simulink model "Control_Law_1e"  (R2020b)
settings: Solver=FixedStepDiscrete  StartTime=0.0  StopTime=60  FixedStep=dt  RelTol=1e-3
InitFcn:
  | clear
  | clc
  | 
  | dtsim = 0.1;
  | dt =0.005;
  | dtdata = 0.01;
  | dtcontrol = 0.01;
  | 
  | I = [1.01560749 0.00028915 0.00002257; 0.00028915 0.17343628 0.00936307; 0.00002257 0.00936307 1.01561864];
  | 
  | Iinv = I^-1;
  | 
  | % Reaction Wheels
  | 
  | x = cosd(70);
  | y = sqrt(0.5*(1^2-x^2));
  | e1 = [x;y;y];
  | e2 = [x;-y;y];
  | e3 = [x;-y;-y];
  | e4 = [x;y;-y];
  | %e1 = [y;x;y];
  | %e2 = [-y;x;y];
  | %e3 = [-y;-x;y];
  | %e4 = [y;-x;y];
  | e = [e1 e2 e3 e4];
  | 
  | %Reaction Wheels MOI and Ang Vel
  | 
  | Irw = 0.000453158;
  | 
  | w1 =1500*2*pi/60;
  | w2 = 1500*2*pi/60;
  | w3 = -1500*2*pi/60;
  | w4 = -1500*2*pi/60;
  | 
  | alpha_max = 1537.9; %rad/sec^2
  | 
  | Tmax = Irw*alpha_max; % Irw*alpha_max;
  | 
  | %User Input Check
  | 
  | Rt = 170*pi/180;
  | Pt = 10*pi/180;
  | Yt = 170*pi/180;
  | 
  | if Pt > 20*pi/180
  | 
  | error('Input a pitch angle lower that 20 degrees')
  | 
  | end
  | 
  | RPYtarget = [Rt;Pt;Yt];
  | 
  | q_target = [cos(Rt/2)*cos(Pt/2)*cos(Yt/2) -  sin(Rt/2)*sin(Pt/2)*sin(Yt/2);
  |                   sin(Rt/2)*cos(Pt/2)*cos(Yt/2) + cos(Rt/2)*sin(Pt/2)*sin(Yt/2);
  |                  cos(Rt/2)*sin(Pt/2)*cos(Yt/2) -   sin(Rt/2)*cos(Pt/2)*sin(Yt/2);
  |                  cos(Rt/2)*cos(Pt/2)*sin(Yt/2) +  sin(Rt/2)*sin(Pt/2)*cos(Yt/2)];
  | 
  | % Inital Conditions
  | 
  | wo = [0;0;0];
  | ro = [6378;0;0];
  | romag = 6378;
  | mu = 398600;
  | vo = sqrt(mu/romag)*[0;1;0];
  | ho = [0;0;0];
  | 
  | a = 6378;
  | n = sqrt(mu/a^3);
  | 
  | %k1 = (4-2)/3;
  | %k2 = (I(3,3) - I(1,1))/I(2,2);
  | %k3  = (I(2,2) - I(1,1))/I(3,3);
  | 
  | k1 = (I(2,2) - I(3,3))/I(1,1);
  | k2 = (I(2,2) - I(3,3))/I(2,2);
  | k3 = (I(2,2) - I(1,1))/I(3,3);
  | 
  | F = -2*n^2*[4*k1, 0, 0;0, 3*k2, 0; 0, 0, k3];
  | G = n*[0 0 (1-k1);0 0 0;(k3-1) 0 0 ];
  | 
  | Iinv =[1/I(1,1) 0 0; 0 1/I(2,2) 0; 0 0 1/I(3,3)];
  | 
  | A = [zeros(3,3) 0.5*eye(3);F G];
  | B = [zeros(3,3); Iinv];
  | R = eye(3);
  | Rinv = R^-1;
  | 
  | Q_nominal= diag([1,1,1,10,10,10]);
  | S_nominal = icare(A,B,Q_nominal,R);
  | K_nominal = -Rinv*B'*S_nominal;
  | 
  | Q_corrective= diag([1,1,1,10,10,10]);
  | S_corrective = icare(A,B,Q_corrective,R);
  | K_corrective = -Rinv*B'*S_corrective;
  | 
  | Q_yawsweep= diag([1,1,1,10,15,10]);
  | S_yawsweep = icare(A,B,Q_yawsweep,R);
  | K_yawsweep = -Rinv*B'*S_yawsweep;
  | 
  | %Initial Attitude
  | 
  | R = 0*pi/180;
  | P = 0*pi/180;
  | Y =0*pi/180;
  | 
  | RPY = [R; P; Y];
  | 
  | qo = [cos(R/2)*cos(P/2)*cos(Y/2) - sin(R/2)*sin(P/2)*sin(Y/2);
  |          sin(R/2)*cos(P/2)*cos(Y/2) + cos(R/2)*sin(P/2)*sin(Y/2);
  |          cos(R/2)*sin(P/2)*cos(Y/2) - sin(R/2)*cos(P/2)*sin(Y/2);
  |          cos(R/2)*cos(P/2)*sin(Y/2) + sin(R/2)*sin(P/2)*cos(Y/2)];
  | 
  | %Visual Int
  | 
  | myworld = vrworld('SimulinkTest.wrl');
  | open(myworld);
  | 
  | set(0,'Units','pixels');
  | scnsize = get(0,'ScreenSize');
  | 
  | f1 = vrfigure(myworld,scnsize);
StopFcn:
  | close all
  | 
  | %Set default grid axes to be on
  | set(groot,'defaultAxesXGrid','on')
  | set(groot,'defaultAxesYGrid','on')
  | 
  | 
  | %Create RPY subplots
  | figure(1)
  | subplot(1,3,1)
  | movegui('northeast')
  | plot(RPY.time,RPY.signals.values(:,1)*180/pi,'-k')
  | hold on
  | plot([0 RPY.time(end)], [1,1]*(rad2deg(RPYtarget(1))+1),'-r')
  | plot([0 RPY.time(end)], [1,1]*(rad2deg(RPYtarget(1))-1),'-r')
  | xlabel('Time (s)')
  | ylabel('Roll (deg)')
  | xlim([0 RPY.time(end)])
  | 
  | set(gca, 'FontSize', 15)
  | 
  | subplot(1,3,2)
  | plot(RPY.time,RPY.signals.values(:,2)*180/pi,'-k')
  | hold on
  | plot([0 RPY.time(end)],  [1,1]*(rad2deg(RPYtarget(2))+1),'-r')
  | plot([0 RPY.time(end)], [1,1]*(rad2deg(RPYtarget(2))-1),'-r')
  | xlabel('Time (s)')
  | ylabel('Pitch (deg)')
  | xlim([0 RPY.time(end)])
  | 
  | set(gca, 'FontSize', 15)
  | 
  | subplot(1,3,3)
  | plot(RPY.time,RPY.signals.values(:,3)*180/pi,'-k')
  | hold on
  | plot([0 RPY.time(end)],  [1,1]*(rad2deg(RPYtarget(3))+1),'-r')
  | plot([0 RPY.time(end)], [1,1]*(rad2deg(RPYtarget(3))-1),'-r')
  | xlabel('Time (s)')
  | ylabel('Yaw (deg)')
  | xlim([0 RPY.time(end)])
  | 
  | set(gca, 'FontSize', 15)
  | 
  | 
  | %Create Angular Position Plots
  | 
  | MagnitudeAngle = 2*acos(q_target(1))*180/pi;
  | 
  | figure(2)
  | movegui('northwest')
  | 
  | hold on
  | 
  | plot(RPY.time,RPY_Mag,'-k')
  | plot([0 RPY.time(end)],  [1,1]*(MagnitudeAngle+1),'-r')
  | plot([0 RPY.time(end)], [1,1]*(MagnitudeAngle-1),'-r')
  | xlabel('Time (sec)')
  | ylabel('Angle (deg)')
  | xlim([0 RPY.time(end)])
  | title('Angular Position Magnitude')
  | box on
  | 
  | 
  | % Create Motor Torque plot
  | figure(3)
  | movegui('south')
  | 
  | %plot(RPY.time,(Motor_Torques.signals.values(1,:)/Tmax)*100,RPY.time,(Motor_Torques.signals.values(2,:)/Tmax)*100,RPY.time,(Motor_Torques.signals.values(3,:)/Tmax)*100,RPY.time,(Motor_Torques.signals.values(4,:)/Tmax)*100)
  | plot(RPY.time,Motor_Torques.signals.values(1,:),RPY.time,Motor_Torques.signals.values(2,:),RPY.time,Motor_Torques.signals.values(3,:),RPY.time,Motor_Torques.signals.values(4,:))
  | xlabel('Time (s)')
  | %ylabel('Torque Percentage (%)')
  | ylabel('Torque (Nm)')
  | title('Motor Torques')
  | legend('Top Motor','Right Motor','Left Motor','Bottom Motor')
  | 
  | 
  | %Create Angular Speed plot
  | figure(4)
  | movegui('southwest')
  | 
  | wmag = sqrt(wvec.signals.values(1,:).^2+wvec.signals.values(2,:).^2+wvec.signals.values(3,:).^2)*180/pi;
  | hold on
  | plot(RPY.time,wmag)
  | plot(RPY.time,0.25.*ones(numel(RPY.time),1))
  | %plot(RPY.time,60*ones(numel(RPY.time),1))
  | xlabel('Time (s)')
  | ylabel('Angular Speed (deg/s)')
  | ylim([-0.5, 20])
  | xlim([0 RPY.time(end)])
  | title('Angular Speed Magnitude')
  | legend('System Angluar Speed', '0.25 deg/s')
  | grid on
  | 
  | 
  | %Create RPY Error plot
  | figure(5)
  | movegui('southeast')
  | hold on
  | plot(RPYerror.time(:,1)', RPYerror.signals.values(:,1), RPYerror.time(:,1)', RPYerror.signals.values(:,2), RPYerror.time(:,1)', RPYerror.signals.values(:,3))
  | plot(RPYerror.time(:,1)', zeros(length(RPYerror.time),1), '--')
  | xlabel('Time (s)')
  | ylabel('Error (°)')
  | title('RPY Error')
  | legend('Roll Error', 'Pitch Error', 'Yaw Error', 'Zero Error')
  | 
  | 
  | %Create Controller Type plot
  | figure(6)
  | movegui('north')
  | 
  | plot(controllerMode.time(:,1)', controllerMode.signals.values)
  | xlabel('Time (s)')
  | ylabel('Controller ID Tag')
  | title('LQR Control Mode vs Time')
  | ylim([0 4])
  | yticks([1,2,3])
undefined symbols (not defined in the file): DiscIntNeverNeededParam
libraries: cstblocks x4, vrlib x2, dspinverses x1, simulink x1, dspmtrx3 x1
settings Model: Creator=lewisbreslin  LastModifiedBy=bnich
settings DataIOCC: ReturnWorkspaceOutputs=off
settings DebuggingCC: ArithmeticOperatorsInVariantConditions=warning
settings SFSimCC: SimUseLocalCustomCode=off  CustomCodeUndefinedFunction=UseInterfaceOnly
settings RTWCC: RTWUseLocalCustomCode=off
settings CodeAppCC: StateflowObjectComments=on

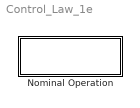
== system Control_Law_1e ==
  "Nominal Operation " : Subsystem  TreatAsAtomicUnit=on

== system Control_Law_1e/Nominal Operation  ==
  1 : RateTransition  InitialCondition=qo  OutPortSampleTime=dtcontrol
  Constant : Constant  Value=q_target
  Controller : Subsystem
  Filter : Subsystem
  Motor Control : Subsystem
  Rate Transition 1 : RateTransition  InitialCondition=qo  OutPortSampleTime=dtsim
  Rate Transition2 : RateTransition  InitialCondition=wo  OutPortSampleTime=dtcontrol
  Rate Transition3 : RateTransition  OutPortSampleTime=dt
  Rate Transition4 : RateTransition  InitialCondition=qo  OutPortSampleTime=dtdata
  VR Sink : vrlib/VR Sink  InstantiateOnLoad=on  SampleTime=0.1  ViewEnable=on  RemoteChange=off  RemoteView=off  FieldsWritten=Phoenix.rotation.4.1.1.double  WorldFileName=SimulinkTest.wrl  AutoView=off  VideoDimensions=[]  AllowVariableSize=off
  Vehicle Dynamics : Subsystem
  q to RPY : Subsystem
  "q to e, phi " : Subsystem
  qerror : Subsystem
  wires:
  Rate Transition4/1 -> q to RPY/1(q)
  Rate Transition3/1 -> Vehicle Dynamics/1(Torque)
  Controller/1(T) -> Motor Control/1(T), Rate Transition3/1
  Rate Transition 1/1 -> "q to e, phi "/1(q)
  Constant/1 -> qerror/1(q_target)
  Rate Transition2/1 -> Controller/5(w)
  Vehicle Dynamics/1(q) -> Rate Transition 1/1, 1/1, Rate Transition4/1
  Vehicle Dynamics/2(w) -> Rate Transition2/1  "w"
  Filter/1(q_observed) -> qerror/2(q_observed)
  1/1 -> Filter/1(In1)
  Motor Control/1(Ho) -> Vehicle Dynamics/2("ho ")
  qerror/2(yawErrorAbs) -> Controller/2(yawErrorAbs)
  qerror/1(qerror) -> Controller/1(qerror)
  qerror/4(q_obs) -> Controller/4(q_obs)
  "q to e, phi "/1("e, phi") -> VR Sink/1
  qerror/3(rollErrorAbs) -> Controller/3(rollErrorAbs)

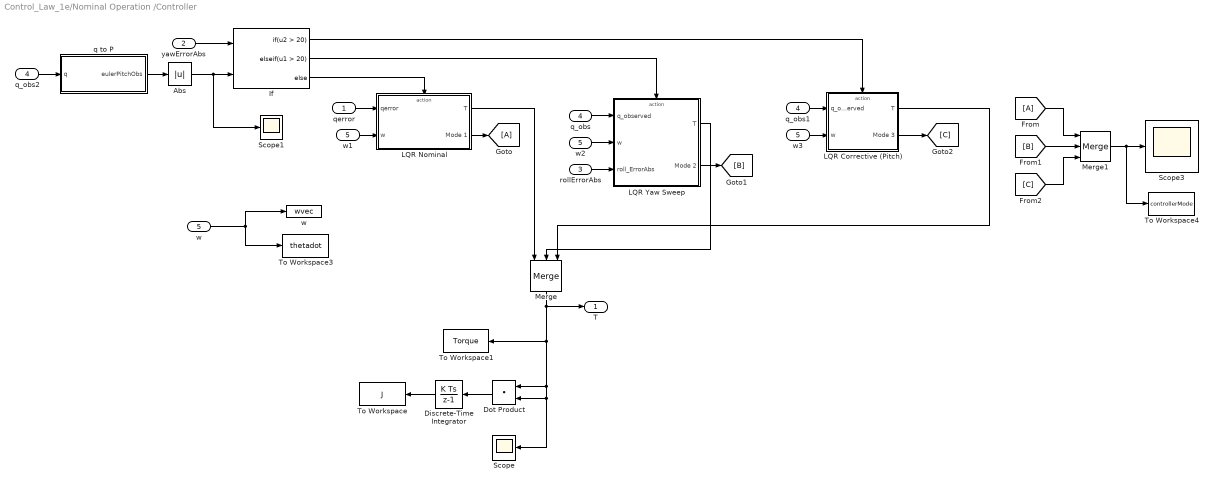
== system Control_Law_1e/Nominal Operation /Controller ==
  qerror : Inport
  yawErrorAbs : Inport  Port=2
  rollErrorAbs : Inport  Port=3
  q_obs : Inport  Port=4
  w : Inport  Port=5
  Abs : Abs
  Discrete-Time Integrator : DiscreteIntegrator  InitialCondition=[0;0;0]  SampleTime=-1  ICPrevOutput=DiscIntNeverNeededParam  ICPrevScaledInput=DiscIntNeverNeededParam
  Dot Product : DotProduct  InputSameDT=on  OutDataTypeStr=Inherit: Inherit via internal rule
  If : If  NumInputs=2  IfExpression=u2 > 20  ElseIfExpressions=u1 > 20
  LQR Corrective (Pitch) : Subsystem
  LQR Nominal : Subsystem  TreatAsAtomicUnit=on
  LQR Yaw Sweep : Subsystem
  Merge : Merge  Inputs=3
  Merge1 : Merge  Inputs=3
  Scope : Scope
  Scope1 : Scope
  Scope3 : Scope
  To Workspace : ToWorkspace  VariableName=J  SampleTime=-1
  To Workspace1 : ToWorkspace  VariableName=Torque  SaveFormat=Structure With Time  SampleTime=-1
  To Workspace3 : ToWorkspace  VariableName=thetadot  SaveFormat=Structure With Time  SampleTime=-1
  To Workspace4 : ToWorkspace  VariableName=controllerMode  SaveFormat=Structure With Time  SampleTime=-1
  q to P : Subsystem
  q_obs1 : InportShadow  Port=4
  q_obs2 : InportShadow  Port=4
  "w " : ToWorkspace  VariableName=wvec  SaveFormat=Structure With Time  SampleTime=-1
  w1 : InportShadow  Port=5
  w2 : InportShadow  Port=5
  w3 : InportShadow  Port=5
  T : Outport
  wires:
  yawErrorAbs/1 -> If/1
  If/3 -> LQR Nominal/Action
  qerror/1 -> LQR Nominal/1(qerror)
  If/1 -> LQR Corrective (Pitch)/Action
  Discrete-Time Integrator/1 -> To Workspace/1
  Merge/1 -> T/1, Scope/1, Dot Product/2, Dot Product/1, To Workspace1/1
  Dot Product/1 -> Discrete-Time Integrator/1
  w/1 -> "w "/1, To Workspace3/1
  q_obs1/1 -> LQR Corrective (Pitch)/1(q_observed)
  q_obs/1 -> LQR Yaw Sweep/1(q_observed)
  q to P/1(eulerPitchObs) -> Abs/1
  If/2 -> LQR Yaw Sweep/Action
  LQR Nominal/1(T) -> Merge/1
  LQR Yaw Sweep/1(T) -> Merge/2
  LQR Corrective (Pitch)/1(T) -> Merge/3
  LQR Nominal/2(Mode 1) -> [A]
  LQR Yaw Sweep/2(Mode 2) -> [B]
  LQR Corrective (Pitch)/2(Mode 3) -> [C]
  [B] -> Merge1/2
  [A] -> Merge1/1
  [C] -> Merge1/3
  Merge1/1 -> To Workspace4/1, Scope3/1
  w3/1 -> LQR Corrective (Pitch)/2(w)
  w2/1 -> LQR Yaw Sweep/2(w)
  w1/1 -> LQR Nominal/2(w)
  q_obs2/1 -> q to P/1(q)
  Abs/1 -> Scope1/1, If/2
  rollErrorAbs/1 -> LQR Yaw Sweep/3(roll_ErrorAbs)

== system Control_Law_1e/Nominal Operation /Filter ==
  In1 : Inport
  Constant{,1..3} (4 alike) : Constant  Value=0.5
  Demux : Demux
  Discrete Varying Lowpass{,1..3} (4 alike) : cstblocks/Linear Parameter Varying/Discrete Varying Lowpass  N=2  w0=0  Ts=dtcontrol
      settings: SourceProductBaseCode=CT
  Mux : Mux
  q_observed : Outport
  wires:
  In1/1 -> Demux/1
  Demux/1 -> Discrete Varying Lowpass/1
  Constant/1 -> Discrete Varying Lowpass/2
  Constant1/1 -> Discrete Varying Lowpass1/2
  Demux/2 -> Discrete Varying Lowpass1/1
  Constant2/1 -> Discrete Varying Lowpass2/2
  Demux/3 -> Discrete Varying Lowpass2/1
  Constant3/1 -> Discrete Varying Lowpass3/2
  Demux/4 -> Discrete Varying Lowpass3/1
  Discrete Varying Lowpass/1 -> Mux/1
  Discrete Varying Lowpass1/1 -> Mux/2
  Discrete Varying Lowpass2/1 -> Mux/3
  Discrete Varying Lowpass3/1 -> Mux/4
  Mux/1 -> q_observed/1

== system Control_Law_1e/Nominal Operation /Motor Control ==
  T : Inport
  Actuator : Subsystem
  Motor control : Subsystem
  Ho : Outport
  wires:
  T/1 -> Actuator/1(Torque)
  Actuator/2(alpha_RW) -> Motor control/2(alpha_RW)
  Motor control/1(Ho) -> Ho/1
  Actuator/1(Irw*e) -> Motor control/1(Irw*e)

== system Control_Law_1e/Nominal Operation /Vehicle Dynamics ==
  note: [0;0;0]
  Torque : Inport
  "ho " : Inport  Port=2
  0;wo] : Memory  InitialCondition=[0;0;0;wo]  InheritSampleTime=on
  Demux : Demux  Outputs=[3;3]
  Difference : simulink/Discrete/Difference  ICPrevInput=[0;0;0]  OutMin=[]  OutMax=[]  OutDataType=fixdt(1, 16)  OutScaling=2^-10  DoSatur=off
  Discrete-Time Integrator : DiscreteIntegrator  IntegratorMethod=Integration: Trapezoidal  gainval=1  InitialConditionSource=external  SampleTime=dt  ICPrevOutput=DiscIntNeverNeededParam  ICPrevScaledInput=DiscIntNeverNeededParam
  Moment Of Inertia Inverse : Constant  Value=Iinv
  "Moment Of inertia " : Constant  Value=I
  Mux : Mux  Inputs=[3 3]
  Subsystem : Subsystem
  Subsystem1 : Subsystem
  "[0;wo]" : Constant  Value=[0;0;0;wo]
  qo : Memory  InitialCondition=qo  InheritSampleTime=on
  q : Outport
  w : Outport  Port=2
  wires:
  Torque/1 -> Subsystem/2(Torque)
  Difference/1 -> Subsystem1/2(Beta)
  0;wo]/1 -> Demux/1
  qo/1 -> Subsystem1/1("qo ")
  Mux/1 -> Discrete-Time Integrator/1
  "Moment Of inertia "/1 -> Subsystem/1(MOI)
  "[0;wo]"/1 -> Discrete-Time Integrator/2
  Subsystem1/1("q1 ") -> q/1, qo/1
  Discrete-Time Integrator/1 -> 0;wo]/1
  Demux/1 -> Difference/1
  Demux/2 -> Subsystem/3(w)
  Subsystem/1("w ") -> w/1, Mux/1
  Subsystem/2("wdot ") -> Mux/2
  Moment Of Inertia Inverse/1 -> Subsystem/4(Inv MOI)
  "ho "/1 -> Subsystem/5("ho ")

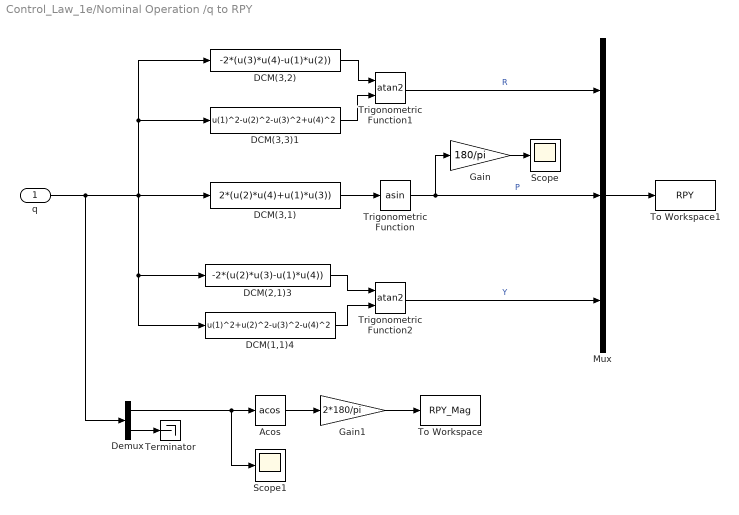
== system Control_Law_1e/Nominal Operation /q to RPY ==
  q : Inport
  Acos : Trigonometry  Operator=acos
  DCM(1,1)4 : Fcn  Expr=u(1)^2+u(2)^2-u(3)^2-u(4)^2
  DCM(2,1)3 : Fcn  Expr=-2*(u(2)*u(3)-u(1)*u(4))
  DCM(3,1) : Fcn  Expr=2*(u(2)*u(4)+u(1)*u(3))
  DCM(3,2) : Fcn  Expr=-2*(u(3)*u(4)-u(1)*u(2))
  DCM(3,3)1 : Fcn  Expr=u(1)^2-u(2)^2-u(3)^2+u(4)^2
  Demux : Demux  Outputs=[1;3]
  Gain : Gain  Gain=180/pi
  Gain1 : Gain  Gain=2*180/pi
  Mux : Mux  Inputs=3
  Scope : Scope
  Scope1 : Scope
  Terminator : Terminator
  To Workspace : ToWorkspace  VariableName=RPY_Mag  SampleTime=dtdata
  To Workspace1 : ToWorkspace  VariableName=RPY  SaveFormat=Structure With Time  SampleTime=dtdata
  Trigonometric Function : Trigonometry  Operator=asin  ApproximationMethod=CORDIC
  Trigonometric Function1 : Trigonometry  Operator=atan2  ApproximationMethod=CORDIC
  Trigonometric Function2 : Trigonometry  Operator=atan2  ApproximationMethod=CORDIC
  wires:
  Trigonometric Function/1 -> Gain/1, Mux/2  "P"
  Trigonometric Function1/1 -> Mux/1  "R"
  DCM(1,1)4/1 -> Trigonometric Function2/2
  DCM(2,1)3/1 -> Trigonometric Function2/1
  DCM(3,3)1/1 -> Trigonometric Function1/2
  DCM(3,2)/1 -> Trigonometric Function1/1
  DCM(3,1)/1 -> Trigonometric Function/1
  Mux/1 -> To Workspace1/1
  Gain/1 -> Scope/1
  Demux/1 -> Acos/1, Scope1/1
  Demux/2 -> Terminator/1
  Acos/1 -> Gain1/1
  Gain1/1 -> To Workspace/1
  Trigonometric Function2/1 -> Mux/3  "Y"
  q/1 -> Demux/1, DCM(3,3)1/1, DCM(3,2)/1, DCM(1,1)4/1, DCM(2,1)3/1, DCM(3,1)/1

== system Control_Law_1e/Nominal Operation /q to e, phi  ==
  q : Inport
  Demux : Demux  Outputs=[1, 3]
  Divide : Product  Inputs=*/
  Gain : Gain  Gain=2
  Mux : Mux  Inputs=2
  Trigonometric Function : Trigonometry  Operator=acos
  Trigonometric Function1 : Trigonometry
  "e, phi" : Outport
  wires:
  Gain/1 -> Mux/2  "phi"
  Trigonometric Function/1 -> Gain/1, Trigonometric Function1/1  "phi/2"
  Divide/1 -> Mux/1  "e"
  Trigonometric Function1/1 -> Divide/2  "sin(phi/2)"
  Mux/1 -> "e, phi"/1
  q/1 -> Demux/1
  Demux/1 -> Trigonometric Function/1  "qo"
  Demux/2 -> Divide/1  "qhat"

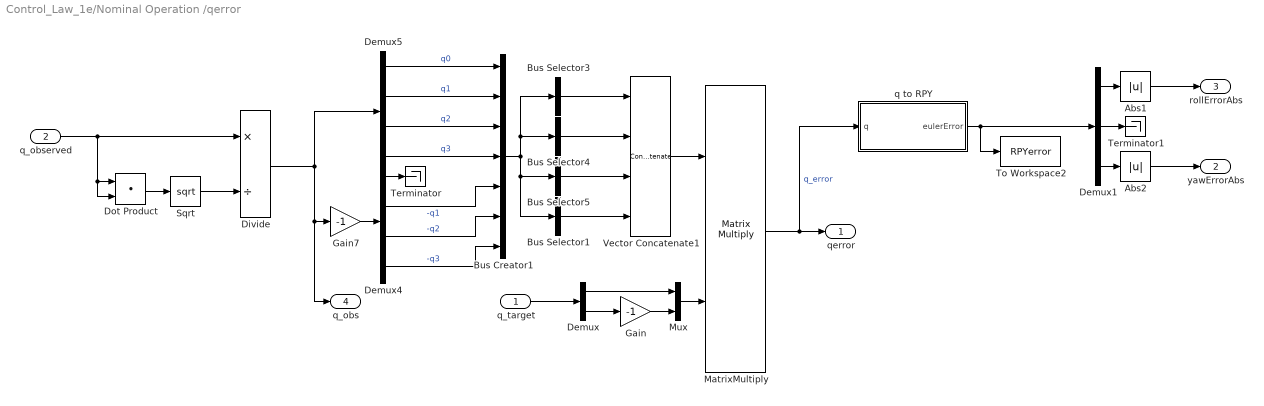
== system Control_Law_1e/Nominal Operation /qerror ==
  q_target : Inport
  q_observed : Inport  Port=2
  Abs1 : Abs
  Abs2 : Abs
  Bus Creator1 : BusCreator  Inputs=7
  Bus Selector1 : BusSelector  OutputSignals=-q3,-q2,q1,q0  OutputAsBus=on
  Bus Selector3 : BusSelector  OutputSignals=q0,q1,q2,q3  OutputAsBus=on
  Bus Selector4 : BusSelector  OutputSignals=-q1,q0,-q3,q2  OutputAsBus=on
  Bus Selector5 : BusSelector  OutputSignals=q2,q3,q0,-q1  OutputAsBus=on
  Demux : Demux  Outputs=[1;3]
  Demux1 : Demux  Outputs=3
  Demux4 : Demux
  Demux5 : Demux
  Divide : Product  Inputs=*/
  Dot Product : DotProduct  InputSameDT=on  OutDataTypeStr=Inherit: Inherit via internal rule
  Gain : Gain  Gain=-1
  Gain7 : Gain  Gain=-1
  MatrixMultiply : Product  Multiplication=Matrix(*)
  Mux : Mux  Inputs=2
  Sqrt : Sqrt  SaturateOnIntegerOverflow=on
  Terminator : Terminator
  Terminator1 : Terminator
  To Workspace2 : ToWorkspace  VariableName=RPYerror  SaveFormat=Structure With Time  SampleTime=-1
  Vector Concatenate1 : Concatenate  NumInputs=4  Mode=Multidimensional array  ConcatenateDimension=2
  q to RPY : Subsystem
  qerror : Outport
  yawErrorAbs : Outport  Port=2
  rollErrorAbs : Outport  Port=3
  q_obs : Outport  Port=4
  wires:
  MatrixMultiply/1 -> q to RPY/1(q), qerror/1  "q_error"
  q_target/1 -> Demux/1
  Demux/1 -> Mux/1
  Demux/2 -> Gain/1
  Gain/1 -> Mux/2
  Mux/1 -> MatrixMultiply/2
  Vector Concatenate1/1 -> MatrixMultiply/1
  Bus Selector1/1 -> Vector Concatenate1/4
  Bus Creator1/1 -> Bus Selector4/1, Bus Selector3/1, Bus Selector5/1, Bus Selector1/1
  Bus Selector4/1 -> Vector Concatenate1/2
  Gain7/1 -> Demux4/1
  Bus Selector5/1 -> Vector Concatenate1/3
  Demux5/1 -> Bus Creator1/1  "q0"
  Demux5/2 -> Bus Creator1/2  "q1"
  Bus Selector3/1 -> Vector Concatenate1/1
  Demux4/3 -> Bus Creator1/6  "-q2"
  Demux5/4 -> Bus Creator1/4  "q3"
  Demux5/3 -> Bus Creator1/3  "q2"
  Demux4/2 -> Bus Creator1/5  "-q1"
  Demux4/4 -> Bus Creator1/7  "-q3"
  Demux4/1 -> Terminator/1
  q_observed/1 -> Dot Product/1, Dot Product/2, Divide/1
  Dot Product/1 -> Sqrt/1
  Sqrt/1 -> Divide/2
  Divide/1 -> Demux5/1, Gain7/1, q_obs/1
  Abs2/1 -> yawErrorAbs/1
  q to RPY/1(eulerError) -> To Workspace2/1, Demux1/1
  Demux1/2 -> Terminator1/1
  Demux1/3 -> Abs2/1
  Abs1/1 -> rollErrorAbs/1
  Demux1/1 -> Abs1/1

== system Control_Law_1e/Nominal Operation /Controller/LQR Corrective (Pitch) ==
  q_observed : Inport
  w : Inport  Port=2
  Action Port : ActionPort  ActionPortLabel=if(u2 > 20)
  Constant : Constant  Value=3
  LQR Corrective (Pitch) : Subsystem
  q_adjustment : Subsystem
  q_observed1 : InportShadow
  qerror : Subsystem
  T : Outport
  Mode 3 : Outport  Port=2
  wires:
  q_adjustment/1(q_adjusted) -> qerror/1(q_adjusted)
  q_observed/1 -> qerror/2(q_observed)
  Constant/1 -> Mode 3/1
  q_observed1/1 -> q_adjustment/1(q_obs)
  qerror/1(qerror) -> LQR Corrective (Pitch)/1(q_error)
  LQR Corrective (Pitch)/1(T) -> T/1
  w/1 -> LQR Corrective (Pitch)/2(w)

== system Control_Law_1e/Nominal Operation /Controller/LQR Nominal ==
  qerror : Inport
  w : Inport  Port=2
  Action Port : ActionPort  ActionPortLabel=else
  Constant : Constant
  LQR Nominal : Subsystem
  T : Outport
  Mode 1 : Outport  Port=2
  wires:
  Constant/1 -> Mode 1/1
  qerror/1 -> LQR Nominal/1(q_error)
  LQR Nominal/1(T) -> T/1
  w/1 -> LQR Nominal/2(w)

== system Control_Law_1e/Nominal Operation /Controller/LQR Yaw Sweep ==
  q_observed : Inport
  w : Inport  Port=2
  roll_ErrorAbs : Inport  Port=3
  Action Port : ActionPort  ActionPortLabel=elseif(u1 > 20 )
  Constant : Constant  Value=q_target
  Constant1 : Constant  Value=2
  Constant2 : Constant  Value=q_target
  If : If  IfExpression=u1 > 20
  If Action Subsystem : Subsystem  TreatAsAtomicUnit=on
  If Action Subsystem1 : Subsystem  TreatAsAtomicUnit=on
  LQR Corrective (Pitch) : Subsystem
  Merge : Merge
  q_observed1 : InportShadow
  T : Outport
  Mode 2 : Outport  Port=2
  wires:
  roll_ErrorAbs/1 -> If/1
  Constant/1 -> If Action Subsystem/1(q_target)
  Constant1/1 -> Mode 2/1
  If/2 -> If Action Subsystem/Action
  LQR Corrective (Pitch)/1(T) -> T/1
  w/1 -> LQR Corrective (Pitch)/1(w)
  If/1 -> If Action Subsystem1/Action
  q_observed/1 -> If Action Subsystem/2(q_observed)
  Merge/1 -> LQR Corrective (Pitch)/2(q_error)
  If Action Subsystem1/1(qerror1) -> Merge/1
  If Action Subsystem/1(qerror1) -> Merge/2
  q_observed1/1 -> If Action Subsystem1/2(q_obs)
  Constant2/1 -> If Action Subsystem1/1(q_target)

== system Control_Law_1e/Nominal Operation /Controller/q to P ==
  q : Inport
  DCM(3,1) : Fcn  Expr=2*(u(2)*u(4)+u(1)*u(3))
  Gain2 : Gain  Gain=180/pi
  Trigonometric Function : Trigonometry  Operator=asin  ApproximationMethod=CORDIC
  eulerPitchObs : Outport
  wires:
  Trigonometric Function/1 -> Gain2/1  "P"
  DCM(3,1)/1 -> Trigonometric Function/1
  q/1 -> DCM(3,1)/1
  Gain2/1 -> eulerPitchObs/1

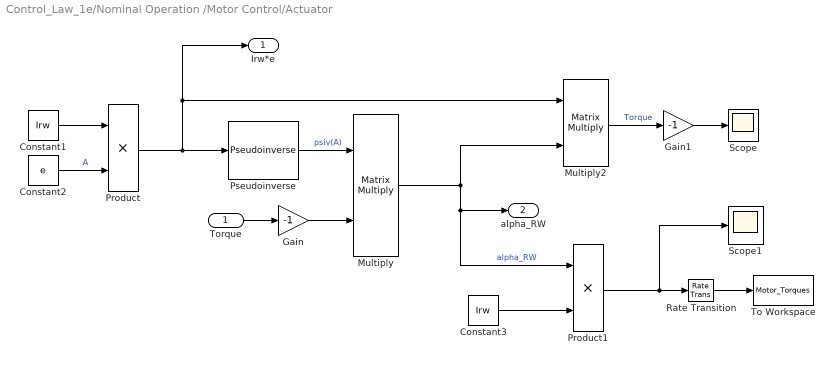
== system Control_Law_1e/Nominal Operation /Motor Control/Actuator ==
  Torque : Inport  PortDimensions=[3,1]
  Constant1 : Constant  Value=Irw
  Constant2 : Constant  Value=e
  Constant3 : Constant  Value=Irw
  Gain : Gain  Gain=-1
  Gain1 : Gain  Gain=-1
  Multiply : Product  Multiplication=Matrix(*)
  Multiply2 : Product  Multiplication=Matrix(*)
  Product : Product
  Product1 : Product
  Pseudoinverse : dspinverses/Pseudoinverse  wanterr=off  SimulateUsing=Interpreted execution
      settings: SourceProductBaseCode=DS
  Rate Transition : RateTransition  InitialCondition=[0;0;0;0]  OutPortSampleTime=dtdata
  Scope : Scope
  Scope1 : Scope
  To Workspace : ToWorkspace  VariableName=Motor_Torques  SaveFormat=Structure With Time  SampleTime=dtdata
  Irw*e : Outport
  alpha_RW : Outport  Port=2
  wires:
  Torque/1 -> Gain/1
  Product/1 -> Irw*e/1, Multiply2/1, Pseudoinverse/1
  Constant1/1 -> Product/1
  Pseudoinverse/1 -> Multiply/1  "psiv(A)"
  Multiply/1 -> Multiply2/2, Product1/1, alpha_RW/1  "alpha_RW"
  Constant2/1 -> Product/2  "A"
  Multiply2/1 -> Gain1/1  "Torque"
  Gain/1 -> Multiply/2
  Gain1/1 -> Scope/1
  Constant3/1 -> Product1/2
  Product1/1 -> Rate Transition/1, Scope1/1
  Rate Transition/1 -> To Workspace/1

== system Control_Law_1e/Nominal Operation /Motor Control/Motor control ==
  Irw*e : Inport
  alpha_RW : Inport  Port=2
  Constant3 : Constant  Value=[w1 ;w2 ;w3 ;w4]  SampleTime=dt
  Discrete-Time Integrator1 : DiscreteIntegrator  IntegratorMethod=Integration: Trapezoidal  InitialConditionSource=external  SampleTime=dt  LimitOutput=on  UpperSaturationLimit=733  LowerSaturationLimit=-733  ICPrevOutput=DiscIntNeverNeededParam  ICPrevScaledInput=DiscIntNeverNeededParam
  Gain : Gain  Gain=60/(2*pi)
  Multiply3 : Product  Multiplication=Matrix(*)
  Scope : Scope
  Ho : Outport
  wires:
  Irw*e/1 -> Multiply3/1  "Irw*e"
  Constant3/1 -> Discrete-Time Integrator1/2
  Multiply3/1 -> Ho/1  "Ho"
  Discrete-Time Integrator1/1 -> Multiply3/2, Gain/1
  alpha_RW/1 -> Discrete-Time Integrator1/1  "alpha_RW"
  Gain/1 -> Scope/1

== system Control_Law_1e/Nominal Operation /Vehicle Dynamics/Subsystem ==
  MOI : Inport
  Torque : Inport  Port=2
  w : Inport  Port=3
  Inv MOI : Inport  Port=4
  "ho " : Inport  Port=5
  Cross Product : vrlib/Utilities/Cross Product
  Product : Product  Multiplication=Matrix(*)
  Product1 : Product  Multiplication=Matrix(*)
  Subtract : Sum  Inputs=-+
  Sum : Sum  Inputs=|++
  "w " : Outport
  "wdot " : Outport  Port=2
  wires:
  Cross Product/1 -> Subtract/1  "wX[I]w"
  Torque/1 -> Subtract/2
  w/1 -> Cross Product/1, "w "/1, Product/2  "w"
  Subtract/1 -> Product1/2
  Product1/1 -> "wdot "/1  "wdot"
  Inv MOI/1 -> Product1/1
  MOI/1 -> Product/1
  "ho "/1 -> Sum/2
  Product/1 -> Sum/1  "[I]*w"
  Sum/1 -> Cross Product/2

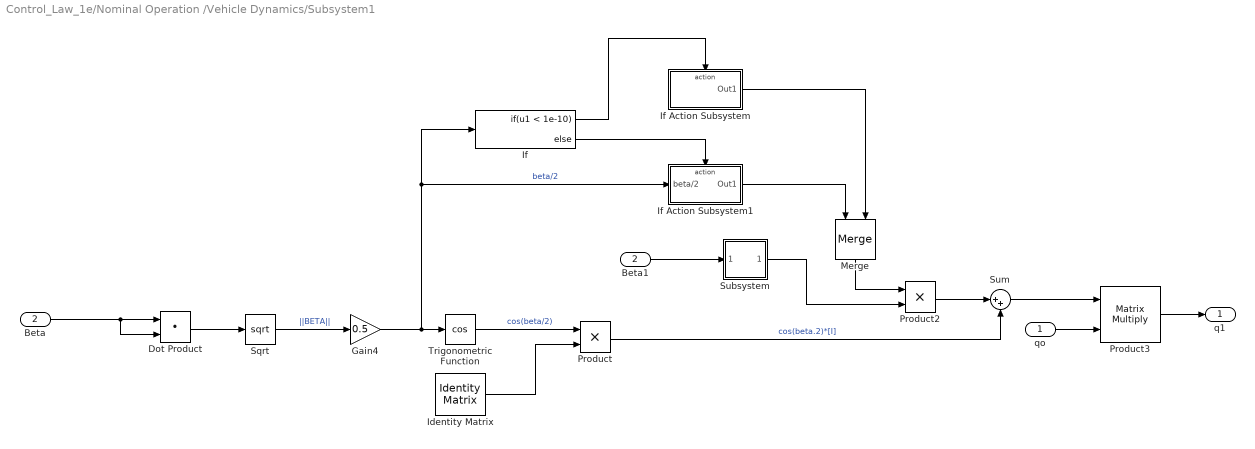
== system Control_Law_1e/Nominal Operation /Vehicle Dynamics/Subsystem1 ==
  "qo " : Inport
  Beta : Inport  Port=2
  Beta1 : InportShadow  Port=2
  Dot Product : DotProduct  InputSameDT=on  OutDataTypeStr=Inherit: Inherit via internal rule
  Gain4 : Gain  Gain=0.5
  Identity Matrix : dspmtrx3/Identity Matrix  Inherit=off  N=4  Ts=1  dataType=double  isSigned=on  wordLen=16  udDataType=sfix(16)  fracBitsMode=Best precision  numFracBits=15  OutDataTypeStr=double  LastOutDataTypeStr=double
  If : If  IfExpression=u1 < 1e-10
  If Action Subsystem : Subsystem  TreatAsAtomicUnit=on
  If Action Subsystem1 : Subsystem  TreatAsAtomicUnit=on
  Merge : Merge
  Product : Product
  Product2 : Product
  Product3 : Product  Multiplication=Matrix(*)
  Sqrt : Sqrt  SaturateOnIntegerOverflow=on
  Subsystem : Subsystem
  Sum : Sum  Inputs=|++
  Trigonometric Function : Trigonometry  Operator=cos
  "q1 " : Outport
  wires:
  Gain4/1 -> If/1, If Action Subsystem1/1(beta/2), Trigonometric Function/1  "beta/2"
  Trigonometric Function/1 -> Product/1  "cos(beta/2)"
  Identity Matrix/1 -> Product/2
  Product/1 -> Sum/2  "cos(beta.2)*[I]"
  Product2/1 -> Sum/1
  Sum/1 -> Product3/1
  "qo "/1 -> Product3/2
  Product3/1 -> "q1 "/1
  Merge/1 -> Product2/1
  Beta/1 -> Dot Product/2, Dot Product/1
  Dot Product/1 -> Sqrt/1
  Sqrt/1 -> Gain4/1  "||BETA||"
  If/1 -> If Action Subsystem/Action
  If/2 -> If Action Subsystem1/Action
  Subsystem/1(RHO) -> Product2/2
  Beta1/1 -> Subsystem/1(In1)
  If Action Subsystem/1(Out1) -> Merge/2
  If Action Subsystem1/1(Out1) -> Merge/1

== system Control_Law_1e/Nominal Operation /qerror/q to RPY ==
  q : Inport
  DCM(1,1)4 : Fcn  Expr=u(1)^2+u(2)^2-u(3)^2-u(4)^2
  DCM(2,1)3 : Fcn  Expr=-2*(u(2)*u(3)-u(1)*u(4))
  DCM(3,1) : Fcn  Expr=2*(u(2)*u(4)+u(1)*u(3))
  DCM(3,2) : Fcn  Expr=-2*(u(3)*u(4)-u(1)*u(2))
  DCM(3,3)1 : Fcn  Expr=u(1)^2-u(2)^2-u(3)^2+u(4)^2
  Gain2 : Gain  Gain=180/pi
  Mux : Mux  Inputs=3
  Trigonometric Function : Trigonometry  Operator=asin  ApproximationMethod=CORDIC
  Trigonometric Function1 : Trigonometry  Operator=atan2  ApproximationMethod=CORDIC
  Trigonometric Function2 : Trigonometry  Operator=atan2  ApproximationMethod=CORDIC
  eulerError : Outport
  wires:
  Trigonometric Function/1 -> Mux/2  "P"
  DCM(1,1)4/1 -> Trigonometric Function2/2
  DCM(2,1)3/1 -> Trigonometric Function2/1
  DCM(3,3)1/1 -> Trigonometric Function1/2
  DCM(3,2)/1 -> Trigonometric Function1/1
  DCM(3,1)/1 -> Trigonometric Function/1
  Trigonometric Function2/1 -> Mux/3  "Y"
  q/1 -> DCM(3,3)1/1, DCM(3,2)/1, DCM(1,1)4/1, DCM(2,1)3/1, DCM(3,1)/1
  Mux/1 -> Gain2/1
  Trigonometric Function1/1 -> Mux/1
  Gain2/1 -> eulerError/1

== system Control_Law_1e/Nominal Operation /Controller/LQR Corrective (Pitch)/LQR Corrective (Pitch) ==
  q_error : Inport
  w : Inport  Port=2
  Constant3 : Constant  Value=K_corrective
  Demux : Demux  Outputs=[1;3]
  Multiply : Product  Multiplication=Matrix(*)
  Mux : Mux  Inputs=2
  Terminator : Terminator
  T : Outport
  wires:
  Constant3/1 -> Multiply/1
  q_error/1 -> Demux/1
  Demux/1 -> Terminator/1
  Mux/1 -> Multiply/2  "xbar"
  Demux/2 -> Mux/1
  w/1 -> Mux/2
  Multiply/1 -> T/1

== system Control_Law_1e/Nominal Operation /Controller/LQR Corrective (Pitch)/q_adjustment ==
  q_obs : Inport
  DCM(1,1)4 : Fcn  Expr=u(1)^2+u(2)^2-u(3)^2-u(4)^2
  DCM(2,1)3 : Fcn  Expr=-2*(u(2)*u(3)-u(1)*u(4))
  DCM(3,1) : Fcn  Expr=2*(u(2)*u(4)+u(1)*u(3))
  DCM(3,2) : Fcn  Expr=-2*(u(3)*u(4)-u(1)*u(2))
  DCM(3,3)1 : Fcn  Expr=u(1)^2-u(2)^2-u(3)^2+u(4)^2
  Gain : Gain  Gain=180/pi
  RPY to q : Subsystem
  Scope : Scope
  Trigonometric Function : Trigonometry  Operator=asin  ApproximationMethod=CORDIC
  Trigonometric Function1 : Trigonometry  Operator=atan2  ApproximationMethod=CORDIC
  Trigonometric Function2 : Trigonometry  Operator=atan2  ApproximationMethod=CORDIC
  q_adjusted : Outport
  wires:
  Trigonometric Function/1 -> Gain/1  "P"
  DCM(1,1)4/1 -> Trigonometric Function2/2
  DCM(2,1)3/1 -> Trigonometric Function2/1
  DCM(3,3)1/1 -> Trigonometric Function1/2
  DCM(3,2)/1 -> Trigonometric Function1/1
  DCM(3,1)/1 -> Trigonometric Function/1
  Gain/1 -> Scope/1
  Trigonometric Function2/1 -> RPY to q/2(Y)  "Y"
  q_obs/1 -> DCM(3,3)1/1, DCM(3,2)/1, DCM(1,1)4/1, DCM(2,1)3/1, DCM(3,1)/1
  RPY to q/1(q_adjusted) -> q_adjusted/1
  Trigonometric Function1/1 -> RPY to q/1(R)  "R"

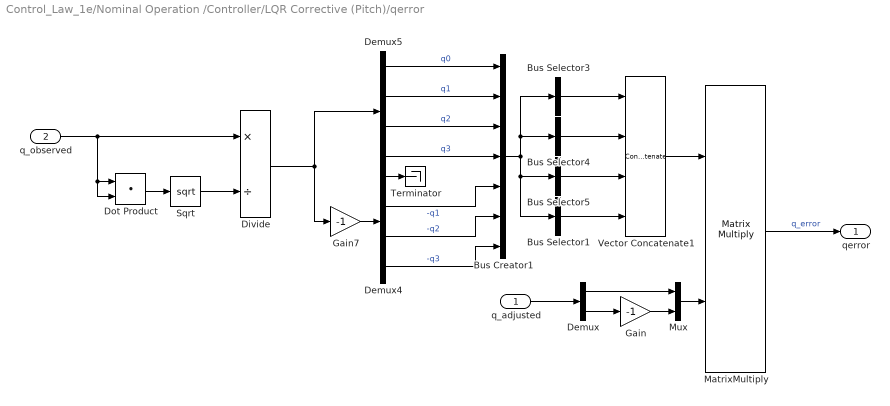
== system Control_Law_1e/Nominal Operation /Controller/LQR Corrective (Pitch)/qerror ==
  q_adjusted : Inport
  q_observed : Inport  Port=2
  Bus Creator1 : BusCreator  Inputs=7
  Bus Selector1 : BusSelector  OutputSignals=-q3,-q2,q1,q0  OutputAsBus=on
  Bus Selector3 : BusSelector  OutputSignals=q0,q1,q2,q3  OutputAsBus=on
  Bus Selector4 : BusSelector  OutputSignals=-q1,q0,-q3,q2  OutputAsBus=on
  Bus Selector5 : BusSelector  OutputSignals=q2,q3,q0,-q1  OutputAsBus=on
  Demux : Demux  Outputs=[1;3]
  Demux4 : Demux
  Demux5 : Demux
  Divide : Product  Inputs=*/
  Dot Product : DotProduct  InputSameDT=on  OutDataTypeStr=Inherit: Inherit via internal rule
  Gain : Gain  Gain=-1
  Gain7 : Gain  Gain=-1
  MatrixMultiply : Product  Multiplication=Matrix(*)
  Mux : Mux  Inputs=2
  Sqrt : Sqrt  SaturateOnIntegerOverflow=on
  Terminator : Terminator
  Vector Concatenate1 : Concatenate  NumInputs=4  Mode=Multidimensional array  ConcatenateDimension=2
  qerror : Outport
  wires:
  MatrixMultiply/1 -> qerror/1  "q_error"
  q_adjusted/1 -> Demux/1
  Demux/1 -> Mux/1
  Demux/2 -> Gain/1
  Gain/1 -> Mux/2
  Mux/1 -> MatrixMultiply/2
  Vector Concatenate1/1 -> MatrixMultiply/1
  Bus Selector1/1 -> Vector Concatenate1/4
  Bus Creator1/1 -> Bus Selector4/1, Bus Selector3/1, Bus Selector5/1, Bus Selector1/1
  Bus Selector4/1 -> Vector Concatenate1/2
  Gain7/1 -> Demux4/1
  Bus Selector5/1 -> Vector Concatenate1/3
  Demux5/1 -> Bus Creator1/1  "q0"
  Demux5/2 -> Bus Creator1/2  "q1"
  Bus Selector3/1 -> Vector Concatenate1/1
  Demux4/3 -> Bus Creator1/6  "-q2"
  Demux5/4 -> Bus Creator1/4  "q3"
  Demux5/3 -> Bus Creator1/3  "q2"
  Demux4/2 -> Bus Creator1/5  "-q1"
  Demux4/4 -> Bus Creator1/7  "-q3"
  Demux4/1 -> Terminator/1
  q_observed/1 -> Dot Product/1, Dot Product/2, Divide/1
  Dot Product/1 -> Sqrt/1
  Sqrt/1 -> Divide/2
  Divide/1 -> Demux5/1, Gain7/1

== system Control_Law_1e/Nominal Operation /Controller/LQR Nominal/LQR Nominal ==
  q_error : Inport
  w : Inport  Port=2
  Constant3 : Constant  Value=K_nominal
  Demux : Demux  Outputs=[1;3]
  Multiply : Product  Multiplication=Matrix(*)
  Mux : Mux  Inputs=2
  Terminator : Terminator
  T : Outport
  wires:
  Constant3/1 -> Multiply/1
  q_error/1 -> Demux/1
  Demux/1 -> Terminator/1
  Mux/1 -> Multiply/2  "xbar"
  Demux/2 -> Mux/1
  w/1 -> Mux/2
  Multiply/1 -> T/1

== system Control_Law_1e/Nominal Operation /Controller/LQR Yaw Sweep/If Action Subsystem ==
  q_target : Inport
  q_observed : Inport  Port=2
  Action Port : ActionPort  ActionPortLabel=else
  q_adjustment : Subsystem
  qerror : Subsystem
  qerror1 : Outport
  wires:
  q_target/1 -> q_adjustment/1(q_target)
  qerror/1(qerror) -> qerror1/1
  q_adjustment/1(q_adjusted) -> qerror/1(q_adjusted)
  q_observed/1 -> qerror/2(q_observed)

== system Control_Law_1e/Nominal Operation /Controller/LQR Yaw Sweep/If Action Subsystem1 ==
  q_target : Inport
  q_obs : Inport  Port=2
  Action Port : ActionPort  ActionPortLabel=if(u1 > 20)
  q_adjustment : Subsystem
  qerror : Subsystem
  qerror1 : Outport
  wires:
  qerror/1(qerror) -> qerror1/1
  q_adjustment/1(q_adjusted) -> qerror/1(q_adjusted)
  q_target/1 -> q_adjustment/1(q_target)
  q_obs/1 -> q_adjustment/2(q_obs), qerror/2(q_observed)

== system Control_Law_1e/Nominal Operation /Controller/LQR Yaw Sweep/LQR Corrective (Pitch) ==
  w : Inport
  q_error : Inport  Port=2
  Constant3 : Constant  Value=K_corrective
  Demux : Demux  Outputs=[1;3]
  Multiply : Product  Multiplication=Matrix(*)
  Mux : Mux  Inputs=2
  Terminator : Terminator
  T : Outport
  wires:
  Constant3/1 -> Multiply/1
  q_error/1 -> Demux/1
  Demux/1 -> Terminator/1
  Mux/1 -> Multiply/2  "xbar"
  Demux/2 -> Mux/1
  w/1 -> Mux/2
  Multiply/1 -> T/1

== system Control_Law_1e/Nominal Operation /Vehicle Dynamics/Subsystem1/If Action Subsystem ==
  Action Port : ActionPort  InitializeStates=reset  ActionPortLabel=if(u1 < 1e-10)
  Constant : Constant  Value=0
  Out1 : Outport
  wires:
  Constant/1 -> Out1/1

== system Control_Law_1e/Nominal Operation /Vehicle Dynamics/Subsystem1/If Action Subsystem1 ==
  beta/2 : Inport
  Action Port : ActionPort  ActionPortLabel=else
  Divide : Product  Inputs=*/
  Trigonometric Function : Trigonometry
  Out1 : Outport
  wires:
  beta/2/1 -> Divide/2, Trigonometric Function/1
  Trigonometric Function/1 -> Divide/1
  Divide/1 -> Out1/1

== system Control_Law_1e/Nominal Operation /Vehicle Dynamics/Subsystem1/Subsystem ==
  In1 : Inport
  Bus Creator : BusCreator  Inputs=7
  Bus Selector : BusSelector  OutputSignals=0,U,V,W  OutputAsBus=on
  Bus Selector1 : BusSelector  OutputSignals=-U,0,-W,V  OutputAsBus=on
  Bus Selector2 : BusSelector  OutputSignals=-V,W,0,-U  OutputAsBus=on
  Bus Selector3 : BusSelector  OutputSignals=-W,-V,U,0  OutputAsBus=on
  Constant : Constant  Value=0
  Demux : Demux  Outputs=3
  Demux2 : Demux  Outputs=3
  Gain : Gain  Gain=-1
  Gain3 : Gain  Gain=0.5
  Vector Concatenate : Concatenate  NumInputs=4  Mode=Multidimensional array  ConcatenateDimension=2
  RHO : Outport
  wires:
  Gain3/1 -> RHO/1  "RHO"
  Demux/1 -> Bus Creator/1  "U"
  Demux/2 -> Bus Creator/2  "V"
  Constant/1 -> Bus Creator/7  "0"
  Bus Selector/1 -> Vector Concatenate/1  "[0;U;V;W]"
  Vector Concatenate/1 -> Gain3/1
  Demux2/2 -> Bus Creator/5  "-V"
  Bus Selector1/1 -> Vector Concatenate/2  "[-U;0;-W;V]"
  In1/1 -> Gain/1, Demux/1
  Bus Selector2/1 -> Vector Concatenate/3  "[-V;W;0;-U]"
  Bus Selector3/1 -> Vector Concatenate/4  "[-W;-V;U;0]"
  Demux/3 -> Bus Creator/3  "W"
  Gain/1 -> Demux2/1  "-U"
  Demux2/3 -> Bus Creator/6  "-W"
  Demux2/1 -> Bus Creator/4  "-U"
  Bus Creator/1 -> Bus Selector3/1, Bus Selector1/1, Bus Selector/1, Bus Selector2/1

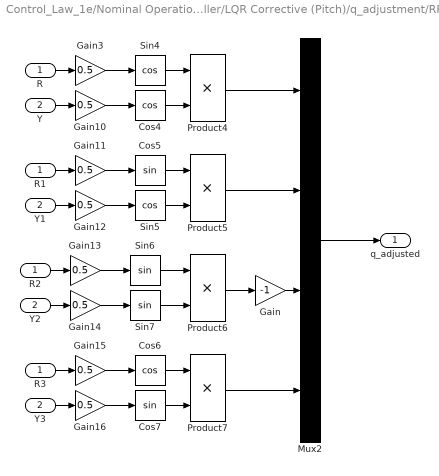
== system Control_Law_1e/Nominal Operation /Controller/LQR Corrective (Pitch)/q_adjustment/RPY to q ==
  R : Inport
  Y : Inport  Port=2
  Cos4 : Trigonometry  Operator=cos
  Cos5 : Trigonometry
  Cos6 : Trigonometry  Operator=cos
  Cos7 : Trigonometry
  Gain : Gain  Gain=-1
  Gain{3,10..16} (8 alike) : Gain  Gain=0.5
  Mux2 : Mux
  Product{4..7} (4 alike) : Product
  R1 : InportShadow
  R2 : InportShadow
  R3 : InportShadow
  Sin4 : Trigonometry  Operator=cos
  Sin5 : Trigonometry  Operator=cos
  Sin6 : Trigonometry
  Sin7 : Trigonometry
  Y1 : InportShadow  Port=2
  Y2 : InportShadow  Port=2
  Y3 : InportShadow  Port=2
  q_adjusted : Outport
  wires:
  Product6/1 -> Gain/1
  Gain11/1 -> Cos5/1
  Cos6/1 -> Product7/1
  R/1 -> Gain3/1
  Cos7/1 -> Product7/2
  Gain16/1 -> Cos7/1
  Y3/1 -> Gain16/1
  Gain14/1 -> Sin7/1
  Cos5/1 -> Product5/1
  Y2/1 -> Gain14/1
  Y/1 -> Gain10/1
  R3/1 -> Gain15/1
  R2/1 -> Gain13/1
  Sin6/1 -> Product6/1
  R1/1 -> Gain11/1
  Gain3/1 -> Sin4/1
  Mux2/1 -> q_adjusted/1
  Gain10/1 -> Cos4/1
  Sin4/1 -> Product4/1
  Gain13/1 -> Sin6/1
  Cos4/1 -> Product4/2
  Y1/1 -> Gain12/1
  Product5/1 -> Mux2/2
  Gain12/1 -> Sin5/1
  Sin7/1 -> Product6/2
  Sin5/1 -> Product5/2
  Gain15/1 -> Cos6/1
  Product4/1 -> Mux2/1
  Product7/1 -> Mux2/4
  Gain/1 -> Mux2/3

== system Control_Law_1e/Nominal Operation /Controller/LQR Yaw Sweep/If Action Subsystem/q_adjustment ==
  q_target : Inport
  DCM(1,1)4 : Fcn  Expr=u(1)^2+u(2)^2-u(3)^2-u(4)^2
  DCM(2,1)3 : Fcn  Expr=-2*(u(2)*u(3)-u(1)*u(4))
  DCM(3,1) : Fcn  Expr=2*(u(2)*u(4)+u(1)*u(3))
  DCM(3,2) : Fcn  Expr=-2*(u(3)*u(4)-u(1)*u(2))
  DCM(3,3)1 : Fcn  Expr=u(1)^2-u(2)^2-u(3)^2+u(4)^2
  Gain : Gain  Gain=180/pi
  RPY to q : Subsystem
  Scope : Scope
  Trigonometric Function : Trigonometry  Operator=asin  ApproximationMethod=CORDIC
  Trigonometric Function1 : Trigonometry  Operator=atan2  ApproximationMethod=CORDIC
  Trigonometric Function2 : Trigonometry  Operator=atan2  ApproximationMethod=CORDIC
  q_adjusted : Outport
  wires:
  Trigonometric Function/1 -> Gain/1  "P"
  DCM(1,1)4/1 -> Trigonometric Function2/2
  DCM(2,1)3/1 -> Trigonometric Function2/1
  DCM(3,3)1/1 -> Trigonometric Function1/2
  DCM(3,2)/1 -> Trigonometric Function1/1
  DCM(3,1)/1 -> Trigonometric Function/1
  Gain/1 -> Scope/1
  Trigonometric Function2/1 -> RPY to q/2(Y)  "Y"
  q_target/1 -> DCM(3,3)1/1, DCM(3,2)/1, DCM(1,1)4/1, DCM(2,1)3/1, DCM(3,1)/1
  RPY to q/1(q_adjusted) -> q_adjusted/1
  Trigonometric Function1/1 -> RPY to q/1(R)  "R"

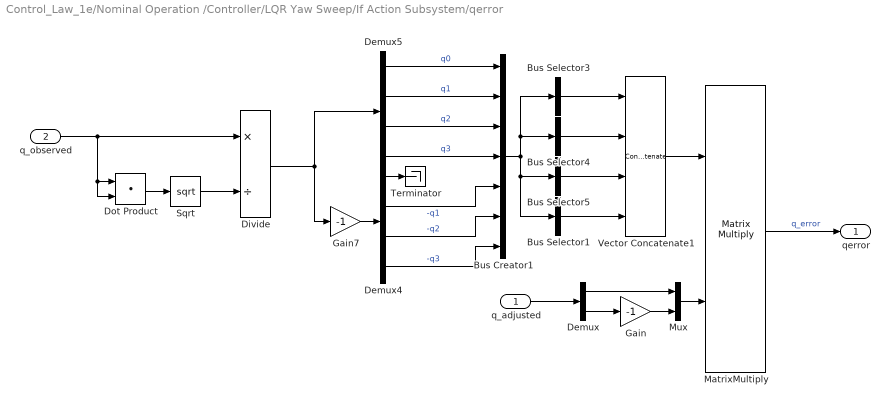
== system Control_Law_1e/Nominal Operation /Controller/LQR Yaw Sweep/If Action Subsystem/qerror ==
  q_adjusted : Inport
  q_observed : Inport  Port=2
  Bus Creator1 : BusCreator  Inputs=7
  Bus Selector1 : BusSelector  OutputSignals=-q3,-q2,q1,q0  OutputAsBus=on
  Bus Selector3 : BusSelector  OutputSignals=q0,q1,q2,q3  OutputAsBus=on
  Bus Selector4 : BusSelector  OutputSignals=-q1,q0,-q3,q2  OutputAsBus=on
  Bus Selector5 : BusSelector  OutputSignals=q2,q3,q0,-q1  OutputAsBus=on
  Demux : Demux  Outputs=[1;3]
  Demux4 : Demux
  Demux5 : Demux
  Divide : Product  Inputs=*/
  Dot Product : DotProduct  InputSameDT=on  OutDataTypeStr=Inherit: Inherit via internal rule
  Gain : Gain  Gain=-1
  Gain7 : Gain  Gain=-1
  MatrixMultiply : Product  Multiplication=Matrix(*)
  Mux : Mux  Inputs=2
  Sqrt : Sqrt  SaturateOnIntegerOverflow=on
  Terminator : Terminator
  Vector Concatenate1 : Concatenate  NumInputs=4  Mode=Multidimensional array  ConcatenateDimension=2
  qerror : Outport
  wires:
  MatrixMultiply/1 -> qerror/1  "q_error"
  q_adjusted/1 -> Demux/1
  Demux/1 -> Mux/1
  Demux/2 -> Gain/1
  Gain/1 -> Mux/2
  Mux/1 -> MatrixMultiply/2
  Vector Concatenate1/1 -> MatrixMultiply/1
  Bus Selector1/1 -> Vector Concatenate1/4
  Bus Creator1/1 -> Bus Selector4/1, Bus Selector3/1, Bus Selector5/1, Bus Selector1/1
  Bus Selector4/1 -> Vector Concatenate1/2
  Gain7/1 -> Demux4/1
  Bus Selector5/1 -> Vector Concatenate1/3
  Demux5/1 -> Bus Creator1/1  "q0"
  Demux5/2 -> Bus Creator1/2  "q1"
  Bus Selector3/1 -> Vector Concatenate1/1
  Demux4/3 -> Bus Creator1/6  "-q2"
  Demux5/4 -> Bus Creator1/4  "q3"
  Demux5/3 -> Bus Creator1/3  "q2"
  Demux4/2 -> Bus Creator1/5  "-q1"
  Demux4/4 -> Bus Creator1/7  "-q3"
  Demux4/1 -> Terminator/1
  q_observed/1 -> Dot Product/1, Dot Product/2, Divide/1
  Dot Product/1 -> Sqrt/1
  Sqrt/1 -> Divide/2
  Divide/1 -> Demux5/1, Gain7/1

== system Control_Law_1e/Nominal Operation /Controller/LQR Yaw Sweep/If Action Subsystem1/q_adjustment ==
  q_target : Inport
  q_obs : Inport  Port=2
  DCM(1,1)4 : Fcn  Expr=u(1)^2+u(2)^2-u(3)^2-u(4)^2
  DCM(2,1)3 : Fcn  Expr=-2*(u(2)*u(3)-u(1)*u(4))
  DCM(3,2) : Fcn  Expr=-2*(u(3)*u(4)-u(1)*u(2))
  DCM(3,3)1 : Fcn  Expr=u(1)^2-u(2)^2-u(3)^2+u(4)^2
  RPY to q : Subsystem
  Trigonometric Function1 : Trigonometry  Operator=atan2  ApproximationMethod=CORDIC
  Trigonometric Function2 : Trigonometry  Operator=atan2  ApproximationMethod=CORDIC
  q_adjusted : Outport
  wires:
  DCM(1,1)4/1 -> Trigonometric Function2/2
  DCM(2,1)3/1 -> Trigonometric Function2/1
  DCM(3,3)1/1 -> Trigonometric Function1/2
  DCM(3,2)/1 -> Trigonometric Function1/1
  Trigonometric Function2/1 -> RPY to q/2(Y)  "Y"
  q_target/1 -> DCM(2,1)3/1, DCM(1,1)4/1
  RPY to q/1(q_adjusted) -> q_adjusted/1
  Trigonometric Function1/1 -> RPY to q/1(R)  "R"
  q_obs/1 -> DCM(3,3)1/1, DCM(3,2)/1

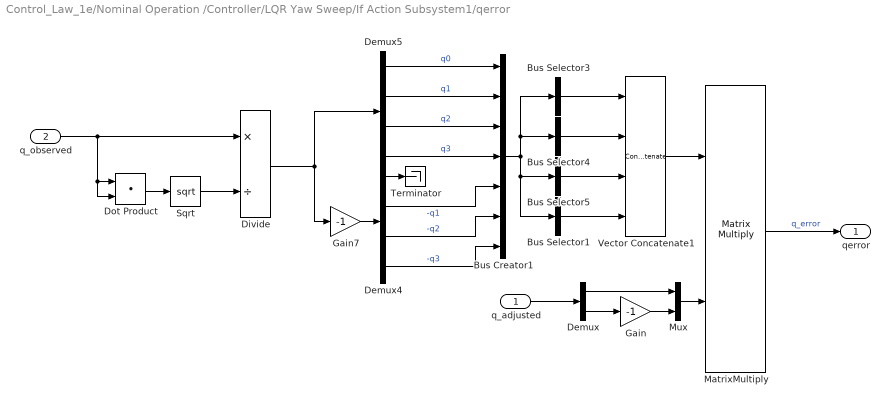
== system Control_Law_1e/Nominal Operation /Controller/LQR Yaw Sweep/If Action Subsystem1/qerror ==
  q_adjusted : Inport
  q_observed : Inport  Port=2
  Bus Creator1 : BusCreator  Inputs=7
  Bus Selector1 : BusSelector  OutputSignals=-q3,-q2,q1,q0  OutputAsBus=on
  Bus Selector3 : BusSelector  OutputSignals=q0,q1,q2,q3  OutputAsBus=on
  Bus Selector4 : BusSelector  OutputSignals=-q1,q0,-q3,q2  OutputAsBus=on
  Bus Selector5 : BusSelector  OutputSignals=q2,q3,q0,-q1  OutputAsBus=on
  Demux : Demux  Outputs=[1;3]
  Demux4 : Demux
  Demux5 : Demux
  Divide : Product  Inputs=*/
  Dot Product : DotProduct  InputSameDT=on  OutDataTypeStr=Inherit: Inherit via internal rule
  Gain : Gain  Gain=-1
  Gain7 : Gain  Gain=-1
  MatrixMultiply : Product  Multiplication=Matrix(*)
  Mux : Mux  Inputs=2
  Sqrt : Sqrt  SaturateOnIntegerOverflow=on
  Terminator : Terminator
  Vector Concatenate1 : Concatenate  NumInputs=4  Mode=Multidimensional array  ConcatenateDimension=2
  qerror : Outport
  wires:
  MatrixMultiply/1 -> qerror/1  "q_error"
  q_adjusted/1 -> Demux/1
  Demux/1 -> Mux/1
  Demux/2 -> Gain/1
  Gain/1 -> Mux/2
  Mux/1 -> MatrixMultiply/2
  Vector Concatenate1/1 -> MatrixMultiply/1
  Bus Selector1/1 -> Vector Concatenate1/4
  Bus Creator1/1 -> Bus Selector4/1, Bus Selector3/1, Bus Selector5/1, Bus Selector1/1
  Bus Selector4/1 -> Vector Concatenate1/2
  Gain7/1 -> Demux4/1
  Bus Selector5/1 -> Vector Concatenate1/3
  Demux5/1 -> Bus Creator1/1  "q0"
  Demux5/2 -> Bus Creator1/2  "q1"
  Bus Selector3/1 -> Vector Concatenate1/1
  Demux4/3 -> Bus Creator1/6  "-q2"
  Demux5/4 -> Bus Creator1/4  "q3"
  Demux5/3 -> Bus Creator1/3  "q2"
  Demux4/2 -> Bus Creator1/5  "-q1"
  Demux4/4 -> Bus Creator1/7  "-q3"
  Demux4/1 -> Terminator/1
  q_observed/1 -> Dot Product/1, Dot Product/2, Divide/1
  Dot Product/1 -> Sqrt/1
  Sqrt/1 -> Divide/2
  Divide/1 -> Demux5/1, Gain7/1

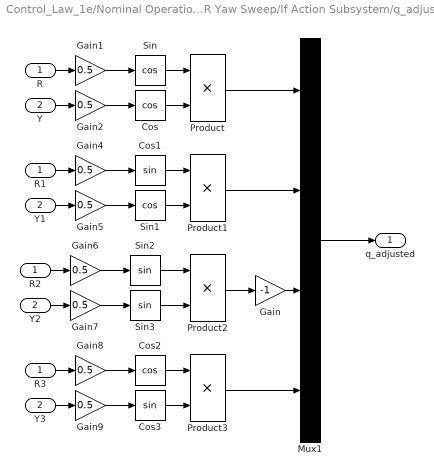
== system Control_Law_1e/Nominal Operation /Controller/LQR Yaw Sweep/If Action Subsystem/q_adjustment/RPY to q ==
  R : Inport
  Y : Inport  Port=2
  Cos : Trigonometry  Operator=cos
  Cos1 : Trigonometry
  Cos2 : Trigonometry  Operator=cos
  Cos3 : Trigonometry
  Gain : Gain  Gain=-1
  Gain{1..2,4..9} (8 alike) : Gain  Gain=0.5
  Mux1 : Mux
  Product{,1..3} (4 alike) : Product
  R1 : InportShadow
  R2 : InportShadow
  R3 : InportShadow
  Sin : Trigonometry  Operator=cos
  Sin1 : Trigonometry  Operator=cos
  Sin2 : Trigonometry
  Sin3 : Trigonometry
  Y1 : InportShadow  Port=2
  Y2 : InportShadow  Port=2
  Y3 : InportShadow  Port=2
  q_adjusted : Outport
  wires:
  Gain2/1 -> Cos/1
  Sin/1 -> Product/1
  Sin3/1 -> Product2/2
  Sin1/1 -> Product1/2
  Mux1/1 -> q_adjusted/1
  Cos/1 -> Product/2
  Sin2/1 -> Product2/1
  Gain8/1 -> Cos2/1
  Cos1/1 -> Product1/1
  Gain6/1 -> Sin2/1
  Product3/1 -> Mux1/4
  Product/1 -> Mux1/1
  Gain5/1 -> Sin1/1
  Gain9/1 -> Cos3/1
  Gain4/1 -> Cos1/1
  Cos2/1 -> Product3/1
  Product1/1 -> Mux1/2
  Gain7/1 -> Sin3/1
  Gain1/1 -> Sin/1
  Cos3/1 -> Product3/2
  R1/1 -> Gain4/1
  Y1/1 -> Gain5/1
  R2/1 -> Gain6/1
  Y2/1 -> Gain7/1
  Y3/1 -> Gain9/1
  R3/1 -> Gain8/1
  Y/1 -> Gain2/1
  R/1 -> Gain1/1
  Gain/1 -> Mux1/3
  Product2/1 -> Gain/1

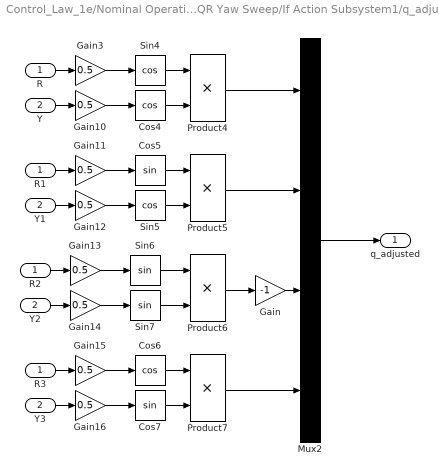
== system Control_Law_1e/Nominal Operation /Controller/LQR Yaw Sweep/If Action Subsystem1/q_adjustment/RPY to q ==
  R : Inport
  Y : Inport  Port=2
  Cos4 : Trigonometry  Operator=cos
  Cos5 : Trigonometry
  Cos6 : Trigonometry  Operator=cos
  Cos7 : Trigonometry
  Gain : Gain  Gain=-1
  Gain{3,10..16} (8 alike) : Gain  Gain=0.5
  Mux2 : Mux
  Product{4..7} (4 alike) : Product
  R1 : InportShadow
  R2 : InportShadow
  R3 : InportShadow
  Sin4 : Trigonometry  Operator=cos
  Sin5 : Trigonometry  Operator=cos
  Sin6 : Trigonometry
  Sin7 : Trigonometry
  Y1 : InportShadow  Port=2
  Y2 : InportShadow  Port=2
  Y3 : InportShadow  Port=2
  q_adjusted : Outport
  wires:
  Product6/1 -> Gain/1
  Gain11/1 -> Cos5/1
  Cos6/1 -> Product7/1
  R/1 -> Gain3/1
  Cos7/1 -> Product7/2
  Gain16/1 -> Cos7/1
  Y3/1 -> Gain16/1
  Gain14/1 -> Sin7/1
  Cos5/1 -> Product5/1
  Y2/1 -> Gain14/1
  Y/1 -> Gain10/1
  R3/1 -> Gain15/1
  R2/1 -> Gain13/1
  Sin6/1 -> Product6/1
  R1/1 -> Gain11/1
  Gain3/1 -> Sin4/1
  Mux2/1 -> q_adjusted/1
  Gain10/1 -> Cos4/1
  Sin4/1 -> Product4/1
  Gain13/1 -> Sin6/1
  Cos4/1 -> Product4/2
  Y1/1 -> Gain12/1
  Product5/1 -> Mux2/2
  Gain12/1 -> Sin5/1
  Sin7/1 -> Product6/2
  Sin5/1 -> Product5/2
  Gain15/1 -> Cos6/1
  Product4/1 -> Mux2/1
  Product7/1 -> Mux2/4
  Gain/1 -> Mux2/3
